simulink model "geyrkhati_khati"  (R2022a)
settings: Solver=VariableStepAuto  StartTime=0.0  StopTime=1000.0  RelTol=1e-3
settings Model: Creator=mamad  LastModifiedBy=mamad

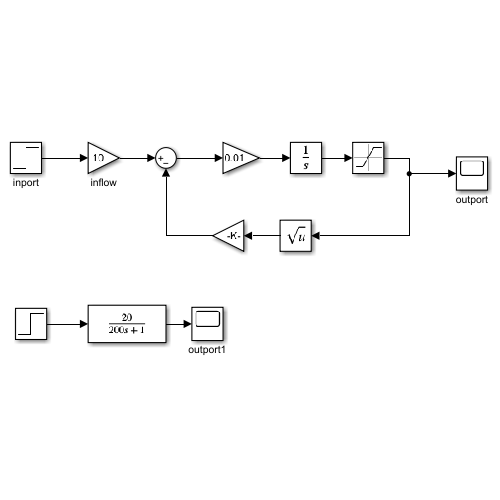
[thumbnail: Simulink's stored preview of the top-level diagram]
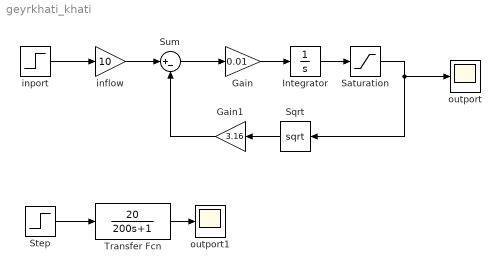
== system geyrkhati_khati ==
  Gain : Gain  Gain=0.01
  Gain1 : Gain  Gain=3.16
  Integrator : Integrator
  Saturation : Saturate  UpperLimit=10  LowerLimit=0
  Sqrt : Sqrt
  Step : Step  SampleTime=0
  Sum : Sum  Inputs=|+-
  Transfer Fcn : TransferFcn  Numerator=[20]  Denominator=[200 1]
  inflow : Gain  Gain=10
  inport : Step  SampleTime=0
  outport : Scope
  outport1 : Scope
  wires:
  inport/1 -> inflow/1
  inflow/1 -> Sum/1
  Sum/1 -> Gain/1
  Gain/1 -> Integrator/1
  Sqrt/1 -> Gain1/1
  Gain1/1 -> Sum/2
  Integrator/1 -> Saturation/1
  Saturation/1 -> outport/1, Sqrt/1
  Step/1 -> Transfer Fcn/1
  Transfer Fcn/1 -> outport1/1
